simulink model "TorqueVect"  (R2022a)
settings: Solver=VariableStepAuto  StartTime=0.0  StopTime=32  RelTol=1e-3
PreLoadFcn:
  | run('Parameters\FSE_Parameters.m')
undefined symbols (not defined in the file): BRegenEnabledButton, canChannel, CyalphaLookUp, efficiency, Fz_curve, Fz_scaling_long, gearR, izz, jw, Kd, kd, Ki, ki, Kp, kp, l_f, l_r, lambda, m, Mz_max, N, N_lat, N_long, P_max, pid_kd_lat, pid_kd_long, pid_ki_lat, pid_ki_long, pid_kp_lat, pid_kp_long, R_max, rw, steerR, T_i_max, TC_Decr_Gas, TC_Derivative, TC_Incr_Gas, TC_On, TC_Relay_Off, TC_Relay_On, tireCornerStiffness, Ts, TV_On, TV_Override, velocity_lookup, velocity_lookup_lat, y_ref, yrr_scaling
libraries: simulink x218, slpidlib x135, CarMaker4SL x101, TractionControlLibrary x13, canmsglib x9, canlib x8, TorqueVectoringLibrary x6, simulink_extras x4, PedalConversionLibrary x3, PowerControlLibrary x1
(part 3 of 26)

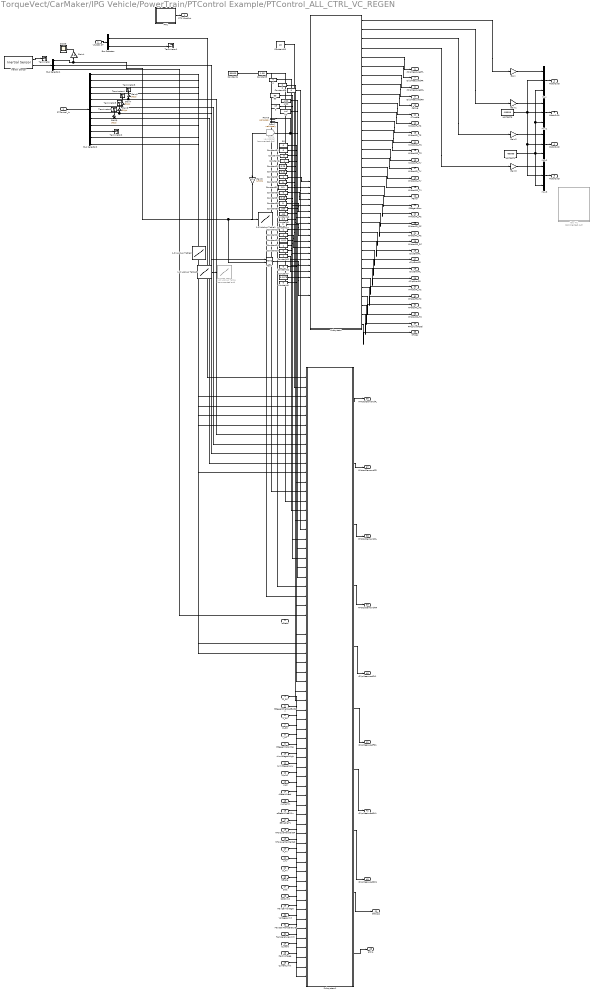
== system TorqueVect/CarMaker/IPG Vehicle/PowerTrain/PTControl Example/PTControl_ALL_CTRL_VC_REGEN ==
  VhclCtrl.PT : Inport
  PTControl_In : Inport  Port=2
  aSteer : Inport  Port=3
  FF_RC : Inport  Port=4
  BRegenEnabledButton : Inport  Port=5
  P_RC : Inport  Port=6
  D_RC : Inport  Port=7
  I_RC : Inport  Port=8
  MRegenMotorMax : Inport  Port=9
  rLimitRegenHigh : Inport  Port=10
  rLimitRegenLow : Inport  Port=11
  rSplitF : Inport  Port=12
  vLat : Inport  Port=13
  rSteerWheel : Inport  Port=14
  vLongMin : Inport  Port=15
  aSteerWheelMin : Inport  Port=16
  BEnableTV : Inport  Port=17
  NTorqueMaxDeltaF : Inport  Port=18
  NTorqueMaxDeltaR : Inport  Port=19
  P_TV : Inport  Port=20
  I_TV : Inport  Port=21
  D_TV : Inport  Port=22
  NBrake : Inport  Port=23
  Current : Inport  Port=24
  PackVoltage : Inport  Port=25
  CurrentLimit : Inport  Port=26
  SOC : Inport  Port=27
  SOClimit : Inport  Port=28
  MaxCellVoltage : Inport  Port=29
  VoltageLimit : Inport  Port=30
  MaxCellTemperature : Inport  Port=31
  TemperatureLimit : Inport  Port=32
  -20 : Constant  Value=-inf
  -200 : Constant  Value=-200
  1-D Lookup Table : Lookup_n-D  Commented=on  NumberOfTableDimensions=1  BreakpointsForDimension1=[0 5 10 15 20]  Table=[0.3 0.3 0.3 0.3 0.3]  ExtrapMethod=Clip  InternalRulePriority=Speed  RndMeth=Simplest
  1-D Lookup Table1 : Lookup_n-D  NumberOfTableDimensions=1  BreakpointsForDimension1=[-1 -0.75 -0.5 -0.25 0 0.25 0.5 0.75 1]  Table=[0.75 0.65 0.58 0.525 0.5 0.475 0.42 0.3 0.2]  ExtrapMethod=Clip  InternalRulePriority=Speed  RndMeth=Simplest
  1-D Lookup Table2 : Lookup_n-D  NumberOfTableDimensions=1  BreakpointsForDimension1=[0 5 10]  Table=[0.1 0.4 0.4]  ExtrapMethod=Clip  InternalRulePriority=Speed  RndMeth=Simplest
  1-D Lookup Table3 : Lookup_n-D  NumberOfTableDimensions=1  BreakpointsForDimension1=[0 5 10 15 20]  Table=[0.1 0.3 0.42 0.475 0.5]  ExtrapMethod=Clip  InternalRulePriority=Speed  RndMeth=Simplest
  2 : Constant  Value=2
  3 : Constant  Value=inf
  30 : Constant  Value=0
  4 : Constant  Value=4
  80 : Constant  Value=80
  Atan2 : Trigonometry  Operator=atan2
  Bus Selector : BusSelector  OutputSignals=VhclCtrl Gas,VhclCtrl Brake
  Bus Selector1 : BusSelector  OutputSignals=Vel_B x,Vel_B y,Omega_B z
  Bus Selector2 : BusSelector  OutputSignals=PT:Motor.PT:Motor:Trq,PT:Motor.PT:Motor1:Trq,PT:Motor.PT:Motor2:Trq,PT:Motor.PT:Motor3:Trq,PT:Motor.PT:Motor:rotv,PT:Motor.PT:Motor1:rotv,PT:Motor.PT:Motor2:rotv,PT:Motor.PT:Motor3:rotv,PT:PwrSupply:HV1:Pwr,Steer.Driver:Steer:Ang,Steer.Car:SteerAngle:FL,Steer.Car:SteerAngle:FR
  Constant10 : Constant  Value=18
  Constant{6,11,24,27} (4 alike) : Constant
  Constant{3,12,18,26,30..31,34,36} (8 alike) : Constant  Value=0
  Constant14 : Constant  Value=2
  Constant15 : Constant  Value=2
  Constant21 : Constant  Value=4
  Constant22 : Constant  Value=0.25
  Constant23 : Constant  Value=0.01
  Constant33 : Constant  Value=0.25
  Constant35 : Constant  Value=0.1
  Constant37 : Constant  Value=0.15
  Constant38 : Constant  Value=5
  Constant39 : Constant  Value=200
  Constant4 : Constant  Value=80000
  Constant40 : Constant  Value=-60
  Constant5 : Constant  Value=1.05
  Constant7 : Constant  Value=0.1975
  Constant9 : Constant  Value=0.5
  From4 : From  Commented=on  GotoTag=yawVelCar  TagVisibility=global
  Gain{,1..3} (4 alike) : Gain  Gain=1/21
  Gain4 : Gain  Gain=3.6
  Gain5 : Gain  Gain=1/9.81
  Gain{6..9} (4 alike) : Gain  Gain=30/pi
  Inertial Sensor : CarMaker4SL/Sensors/Inertial Sensor  xname=Param_B00  xstime=Continuous
      settings: SourceProductName=CarMaker4SL
  Mux{,1..3} (4 alike) : Mux  Inputs=3
  NOTSET1 : Constant  Value=-99999
  NOTSET3 : Constant  Value=-99999
  New TC : Subsystem  Commented=on
  PTC : Subsystem
  Scope : Scope
  Subsystem : Subsystem
  Subsystem1 : Subsystem
  Terminator{,1..6} (7 alike) : Terminator
  PTC MiscOut : Outport  VectorParamsAs1DForOutWhenUnconnected=off
  MotorOut0 : Outport  Port=2  VectorParamsAs1DForOutWhenUnconnected=off
  MotorOut1 : Outport  Port=3  VectorParamsAs1DForOutWhenUnconnected=off
  MotorOut2 : Outport  Port=4  VectorParamsAs1DForOutWhenUnconnected=off
  MotorOut3 : Outport  Port=5  VectorParamsAs1DForOutWhenUnconnected=off
  rSlipMeasuredFL : Outport  Port=6
  rSlipMeasuredFR : Outport  Port=7
  rSlipMeasuredRL : Outport  Port=8
  rSlipMeasuredRR : Outport  Port=9
  debug : Outport  Port=10
  rThrottle : Outport  Port=11
  MMotorFL_TS : Outport  Port=12
  MMotorFR_TS : Outport  Port=13
  MMotorRL_TS : Outport  Port=14
  MMotorRR_TS : Outport  Port=15
  MMotorFL_TV : Outport  Port=16
  MMotorFR_TV : Outport  Port=17
  MMotorRL_TV : Outport  Port=18
  MMotorRR_TV : Outport  Port=19
  PError : Outport  Port=20
  PRegenError : Outport  Port=21
  MMotorFL_PC : Outport  Port=22
  MMotorFR_PC : Outport  Port=23
  MMotorRL_PC : Outport  Port=24
  MMotorRR_PC : Outport  Port=25
  rSlipErrorFL : Outport  Port=26
  rSlipErrorFR : Outport  Port=27
  rSlipErrorRL : Outport  Port=28
  rSlipErrorRR : Outport  Port=29
  MMotorFL_TC : Outport  Port=30
  MMotorFR_TC : Outport  Port=31
  MMotorRL_TC : Outport  Port=32
  MMotorRR_TC : Outport  Port=33
  PPositiveTotal : Outport  Port=34
  PTotal : Outport  Port=35
  MMotorDemandFL : Outport  Port=36
  MMotorDemandFR : Outport  Port=37
  MMotorDemandRL : Outport  Port=38
  MMotorDemandRR : Outport  Port=39
  rSlipMeasuredFL1 : Outport  Port=40
  rSlipMeasuredFR1 : Outport  Port=41
  rSlipMeasuredRL1 : Outport  Port=42
  rSlipMeasuredRR1 : Outport  Port=43
  debug1 : Outport  Port=44
  aSlip : Outport  Port=45
  wires:
  VhclCtrl.PT/1 -> Bus Selector/1
  PTC/1(PTC MiscOut) -> PTC MiscOut/1
  Inertial Sensor/2 -> Bus Selector1/1
  Bus Selector1/1 -> Subsystem1/24(vLong), Atan2/2, Gain4/1  "<Vel_B x>"
  Inertial Sensor/1 -> Terminator/1
  Mux/1 -> MotorOut0/1
  Mux3/1 -> MotorOut3/1
  Mux2/1 -> MotorOut2/1
  Mux1/1 -> MotorOut1/1
  NOTSET3/1 -> Mux/2, Mux3/2, Mux2/2, Mux1/2
  NOTSET1/1 -> Mux/3, Mux1/3, Mux3/3, Mux2/3  "rotv_trg"
  Gain/1 -> Mux/1
  Gain1/1 -> Mux1/1
  Gain2/1 -> Mux2/1
  Gain3/1 -> Mux3/1
  Gain4/1 -> Scope/1
  3/1 -> Subsystem1/20(rLimitThrottleHigh)
  Constant6/1 -> Subsystem1/33(FF_TC)
  PTControl_In/1 -> Bus Selector2/1
  Subsystem/1(MMotorDemandFL) -> Gain/1
  Subsystem/2(MMotorDemandFR) -> Gain1/1
  Subsystem/3(MMotorDemandRL) -> Gain2/1
  Subsystem/4(MMotorDemandRR) -> Gain3/1
  Bus Selector2/1 -> Subsystem1/4(MMotorFR)  "<PT:Motor:Trq>"
  Bus Selector2/2 -> Subsystem1/3(MMotorFL)  "<PT:Motor1:Trq>"
  Bus Selector2/3 -> Subsystem1/5(MMotorRL)  "<PT:Motor2:Trq>"
  Bus Selector2/4 -> Subsystem1/6(MMotorRR)  "<PT:Motor3:Trq>"
  Bus Selector2/9 -> Subsystem1/11(PMeasured)  "<PT:PwrSupply:HV1:Pwr>"
  Constant11/1 -> Subsystem/43(BTVEnable)
  Constant12/1 -> Subsystem1/25(BEnableTC)
  Bus Selector2/5 -> Subsystem1/7(nMotorFL), Gain6/1  "<PT:Motor:rotv>"
  Bus Selector2/6 -> Subsystem1/8(nMotorFR), Gain7/1  "<PT:Motor1:rotv>"
  Bus Selector2/7 -> Subsystem1/9(nMotorRL), Gain8/1  "<PT:Motor2:rotv>"
  Bus Selector2/8 -> Subsystem1/10(nMotorRR), Gain9/1  "<PT:Motor3:rotv>"
  Constant14/1 -> Subsystem/37(NTorqueMaxDeltaF)
  Constant15/1 -> Subsystem/38(NTorqueMaxDeltaR)
  Bus Selector2/10 -> Terminator2/1  "<Driver:Steer:Ang>"
  Constant18/1 -> Subsystem/42(BRegenEnable)
  Constant23/1 -> Subsystem/40(I_TV)
  Constant24/1 -> Subsystem/41(D_TV)
  Constant21/1 -> Subsystem/39(P_TV)
  Bus Selector/2 -> Terminator1/1  "<VhclCtrl Brake>"
  Bus Selector1/2 -> Atan2/1  "<Vel_B y>"
  Bus Selector/1 -> Subsystem1/1(rThrottlePedal)  "<VhclCtrl Gas>"
  Bus Selector1/3 -> Subsystem1/26(nYaw)  "<Omega_B z>"
  Bus Selector2/11 -> Subsystem1/30(aSteerFL)  "<Car:SteerAngle:FL>"
  Bus Selector2/12 -> Subsystem1/29(aSteerFR)  "<Car:SteerAngle:FR>"
  Subsystem/6(rSlipMeasuredFR) -> rSlipMeasuredFR/1
  Subsystem/25(rSlipErrorFL) -> rSlipErrorFL/1
  Subsystem/30(MMotorFR_TC) -> MMotorFR_TC/1
  Atan2/1 -> Subsystem/44(aSlip)
  Subsystem/14(MMotorRR_TS) -> MMotorRR_TS/1
  Subsystem/28(rSlipErrorRR) -> rSlipErrorRR/1
  Subsystem/31(MMotorRL_TC) -> MMotorRL_TC/1
  Subsystem/26(rSlipErrorFR) -> rSlipErrorFR/1
  Subsystem/19(PError) -> PError/1
  Subsystem/23(MMotorRL_PC) -> MMotorRL_PC/1
  Subsystem/16(MMotorFR_TV) -> MMotorFR_TV/1
  Subsystem/24(MMotorRR_PC) -> MMotorRR_PC/1
  Subsystem/29(MMotorFL_TC) -> MMotorFL_TC/1
  Subsystem/32(MMotorRR_TC) -> MMotorRR_TC/1
  Subsystem/8(rSlipMeasuredRR) -> rSlipMeasuredRR/1
  Subsystem/12(MMotorFR_TS) -> MMotorFR_TS/1
  Subsystem/34(PTotal) -> PTotal/1
  Subsystem/10(rThrottle) -> rThrottle/1
  Subsystem/21(MMotorFL_PC) -> MMotorFL_PC/1
  Subsystem/15(MMotorFL_TV) -> MMotorFL_TV/1
  Constant4/1 -> Subsystem1/13(PLimit)
  Subsystem/7(rSlipMeasuredRL) -> rSlipMeasuredRL/1
  Subsystem/20(PRegenError) -> PRegenError/1
  Subsystem/22(MMotorFR_PC) -> MMotorFR_PC/1
  Subsystem/9(debug) -> debug/1
  Subsystem/5(rSlipMeasuredFL) -> rSlipMeasuredFL/1
  Subsystem/18(MMotorRR_TV) -> MMotorRR_TV/1
  Constant5/1 -> Subsystem1/14(FF_PC)
  Constant10/1 -> Subsystem1/2(MMotorMax)
  Subsystem/13(MMotorRL_TS) -> MMotorRL_TS/1
  Subsystem/11(MMotorFL_TS) -> MMotorFL_TS/1
  Subsystem/27(rSlipErrorRL) -> rSlipErrorRL/1
  Subsystem/17(MMotorRL_TV) -> MMotorRL_TV/1
  4/1 -> Subsystem1/15(P_PC)
  Subsystem/33(PPositiveTotal) -> PPositiveTotal/1
  2/1 -> Subsystem1/16(D_PC)
  Constant26/1 -> Subsystem1/17(I_PC)
  80/1 -> Subsystem1/18(rLimitHigh)
  -200/1 -> Subsystem1/19(rLimitLow)
  30/1 -> Subsystem1/28(P_TC)
  Constant31/1 -> Subsystem1/31(D_TC)
  Constant30/1 -> Subsystem1/32(I_TC)
  Constant22/1 -> Subsystem1/34(rSlipTargetF)
  Constant33/1 -> Subsystem1/35(rSlipTargetR)
  Constant27/1 -> Subsystem/28(FF_RC)
  Constant34/1 -> Subsystem/29(PRegenLimit)
  Constant35/1 -> Subsystem/30(P_RC)
  Constant36/1 -> Subsystem/31(D_RC)
  Constant37/1 -> Subsystem/32(I_RC)
  Constant38/1 -> Subsystem/33(MRegenMotorMax)
  Constant39/1 -> Subsystem/34(rLimitRegenHigh)
  Constant40/1 -> Subsystem/35(rLimitRegenLow)
  [vehAccelx] -> Subsystem1/22(aLong), Gain5/1
  Constant3/1 -> Subsystem1/12(BMeasuredEnable)
  -20/1 -> Subsystem1/21(rLimitThrottleLow)
  1-D Lookup Table3/1 -> 1-D Lookup Table/1
  Gain5/1 -> 1-D Lookup Table1/1
  Constant7/1 -> Subsystem/47(rWheel)
  Constant9/1 -> Subsystem/36(rSplitF)
  Gain6/1 -> Terminator3/1  "FL RPM"
  Gain8/1 -> Terminator5/1  "RL RPM"
  Gain7/1 -> Terminator4/1  "FR RPM"
  Gain9/1 -> Terminator6/1  "RR RPM"
  [vehAccely] -> Subsystem1/23(aLat)
  MaxCellVoltage/1 -> Subsystem1/58(MaxCellVoltage)
  vLongMin/1 -> Subsystem1/47(vLongMin)
  CurrentLimit/1 -> Subsystem1/64(CurrentLimit)
  NBrake/1 -> Subsystem1/55(NBrake)
  I_RC/1 -> Subsystem1/40(I_RC)
  rSteerWheel/1 -> Subsystem1/46(rSteerWheel)
  Subsystem1/4(MMotorDemandRR) -> MMotorDemandRR/1
  Subsystem1/5(rSlipMeasuredFL) -> rSlipMeasuredFL1/1
  P_RC/1 -> Subsystem1/38(P_RC)
  Current/1 -> Subsystem1/62(Current)
  BRegenEnabledButton/1 -> Subsystem1/37(BRegenEnabledButton)
  Subsystem1/3(MMotorDemandRL) -> MMotorDemandRL/1
  Subsystem1/1(MMotorDemandFL) -> MMotorDemandFL/1
  Subsystem1/7(rSlipMeasuredRL) -> rSlipMeasuredRL1/1
  Subsystem1/2(MMotorDemandFR) -> MMotorDemandFR/1
  rLimitRegenHigh/1 -> Subsystem1/42(rLimitRegenHigh)
  SOC/1 -> Subsystem1/56(SOC)
  VoltageLimit/1 -> Subsystem1/59(VoltageLimit)
  SOClimit/1 -> Subsystem1/57(SOClimit)
  MRegenMotorMax/1 -> Subsystem1/41(MRegenMotorMax)
  rLimitRegenLow/1 -> Subsystem1/43(rLimitRegenLow)
  Subsystem1/8(rSlipMeasuredRR) -> rSlipMeasuredRR1/1
  TemperatureLimit/1 -> Subsystem1/61(TemperatureLimit)
  FF_RC/1 -> Subsystem1/36(FF_RC)
  rSplitF/1 -> Subsystem1/44(rSplitF)
  aSteerWheelMin/1 -> Subsystem1/48(aSteerWheelMin)
  I_TV/1 -> Subsystem1/53(I_TV)
  NTorqueMaxDeltaF/1 -> Subsystem1/50(NTorqueMaxDeltaF)
  Subsystem1/9(debug) -> debug1/1
  Subsystem1/6(rSlipMeasuredFR) -> rSlipMeasuredFR1/1
  NTorqueMaxDeltaR/1 -> Subsystem1/51(NTorqueMaxDeltaR)
  MaxCellTemperature/1 -> Subsystem1/60(MaxCellTemperature)
  D_RC/1 -> Subsystem1/39(D_RC)
  D_TV/1 -> Subsystem1/54(D_TV)
  Subsystem1/10(aSlip) -> aSlip/1
  BEnableTV/1 -> Subsystem1/49(BTorqueVectoringEnable)
  PackVoltage/1 -> Subsystem1/63(PackVoltage)
  vLat/1 -> Subsystem1/45(vLat)
  P_TV/1 -> Subsystem1/52(P_TV)

== system TorqueVect/CarMaker/IPG Vehicle/PowerTrain/PTControl Example/PTControl_ALL_Speedgoat ==
  VhclCtrl.PT : Inport
  PTControl_In : Inport  Port=2
  Gain{,1..3} (4 alike) : Gain  Gain=1/21
  Mux{,1..3} (4 alike) : Mux  Inputs=3
  NOTSET1 : Constant  Value=-99999
  NOTSET3 : Constant  Value=-99999
  New TC : Subsystem  Commented=on
  PTC : Subsystem
  Subsystem : Subsystem
  PTC MiscOut : Outport  VectorParamsAs1DForOutWhenUnconnected=off
  MotorOut0 : Outport  Port=2  VectorParamsAs1DForOutWhenUnconnected=off
  MotorOut1 : Outport  Port=3  VectorParamsAs1DForOutWhenUnconnected=off
  MotorOut2 : Outport  Port=4  VectorParamsAs1DForOutWhenUnconnected=off
  MotorOut3 : Outport  Port=5  VectorParamsAs1DForOutWhenUnconnected=off
  wires:
  PTC/1(PTC MiscOut) -> PTC MiscOut/1
  Mux/1 -> MotorOut0/1
  Mux3/1 -> MotorOut3/1
  Mux2/1 -> MotorOut2/1
  Mux1/1 -> MotorOut1/1
  NOTSET3/1 -> Mux3/2, Mux2/2, Mux1/2, Mux/2
  NOTSET1/1 -> Mux3/3, Mux2/3, Mux/3, Mux1/3  "rotv_trg"
  Gain/1 -> Mux/1
  Gain1/1 -> Mux1/1
  Gain2/1 -> Mux2/1
  Gain3/1 -> Mux3/1
  VhclCtrl.PT/1 -> Subsystem/1(VhclCtrl.PT)
  PTControl_In/1 -> Subsystem/2(PTControl_In)
  Subsystem/1(<PT:Motor:Trq>) -> Gain/1
  Subsystem/2(<PT:Motor1:Trq>) -> Gain1/1
  Subsystem/3(<PT:Motor2:Trq>) -> Gain2/1
  Subsystem/4(<PT:Motor3:Trq>) -> Gain3/1

== system TorqueVect/CarMaker/IPG Vehicle/PowerTrain/PTControl Example/PTControl_In ==
  note: [1:43 PM] Ali (Guest)rTireSlipCombinedXX = sqrt(rTireSlipXX^2 + aTireSlipXX^2)
  Sync_In : Inport
  Add{,1..3} (4 alike) : Sum
  Bus Creator : BusCreator  Inputs=8
  Bus Creator1 : BusCreator  Inputs=4
  Bus Creator2 : BusCreator  Inputs=4
  Bus Creator3 : BusCreator  Inputs=3
  CreateBus PTControl_In : BusCreator  Inputs=4
  Read CM Dict : CarMaker4SL/Read CM Dict  xname=PT.Motor.Trq  xsync=on  xstime=Continuous
  Read CM Dict1 : CarMaker4SL/Read CM Dict  xname=PT.Motor1.Trq  xsync=on  xstime=Continuous
  Read CM Dict10 : CarMaker4SL/Read CM Dict  xname=Vhcl.FR.LongSlip  xsync=on  xstime=Continuous
  Read CM Dict11 : CarMaker4SL/Read CM Dict  xname=Vhcl.RL.LongSlip  xsync=on  xstime=Continuous
  Read CM Dict12 : CarMaker4SL/Read CM Dict  xname=Vhcl.RR.LongSlip  xsync=on  xstime=Continuous
  Read CM Dict13 : CarMaker4SL/Read CM Dict  xname=Driver.Steer.Ang  xsync=on  xstime=Continuous
  Read CM Dict14 : CarMaker4SL/Read CM Dict  xname=Vhcl.FR.LongSlip  xsync=on  xstime=Continuous
  Read CM Dict15 : CarMaker4SL/Read CM Dict  xname=Vhcl.RL.LongSlip  xsync=on  xstime=Continuous
  Read CM Dict16 : CarMaker4SL/Read CM Dict  xname=Vhcl.RR.LongSlip  xsync=on  xstime=Continuous
  Read CM Dict17 : CarMaker4SL/Read CM Dict  xname=Vhcl.FL.LongSlip  xsync=on  xstime=Continuous
  Read CM Dict18 : CarMaker4SL/Read CM Dict  xname=Vhcl.FR.SideSlip  xsync=on  xstime=Continuous
  Read CM Dict19 : CarMaker4SL/Read CM Dict  xname=Vhcl.RL.SideSlip  xsync=on  xstime=Continuous
  Read CM Dict2 : CarMaker4SL/Read CM Dict  xname=PT.Motor2.Trq  xsync=on  xstime=Continuous
  Read CM Dict20 : CarMaker4SL/Read CM Dict  xname=Vhcl.RR.SideSlip  xsync=on  xstime=Continuous
  Read CM Dict21 : CarMaker4SL/Read CM Dict  xname=Vhcl.FL.SideSlip  xsync=on  xstime=Continuous
  Read CM Dict22 : CarMaker4SL/Read CM Dict  xname=Car.SteerAngleFL  xsync=on  xstime=Continuous
  Read CM Dict23 : CarMaker4SL/Read CM Dict  xname=Car.SteerAngleFR  xsync=on  xstime=Continuous
  Read CM Dict24 : CarMaker4SL/Read CM Dict  xname=Car.WFL.Radius  xsync=on  xstime=Continuous
  Read CM Dict3 : CarMaker4SL/Read CM Dict  xname=PT.Motor3.Trq  xsync=on  xstime=Continuous
  Read CM Dict4 : CarMaker4SL/Read CM Dict  xname=PT.Motor.rotv  xsync=on  xstime=Continuous
  Read CM Dict5 : CarMaker4SL/Read CM Dict  xname=PT.Motor1.rotv  xsync=on  xstime=Continuous
  Read CM Dict6 : CarMaker4SL/Read CM Dict  xname=PT.Motor2.rotv  xsync=on  xstime=Continuous
  Read CM Dict7 : CarMaker4SL/Read CM Dict  xname=PT.Motor3.rotv  xsync=on  xstime=Continuous
  Read CM Dict8 : CarMaker4SL/Read CM Dict  xname=PT.PwrSupply.HV1.Pwr  xsync=on  xstime=Continuous
  Read CM Dict9 : CarMaker4SL/Read CM Dict  xname=Vhcl.FL.LongSlip  xsync=on  xstime=Continuous
  Sqrt{,1..3} (4 alike) : Sqrt
  Square{,1..7} (8 alike) : Math  Operator=square
  Terminator : Terminator
  Terminator1 : Terminator
  PTControl_In : Outport  VectorParamsAs1DForOutWhenUnconnected=off
  wires:
  Sync_In/1 -> Read CM Dict2/1, Read CM Dict/1, Read CM Dict1/1, Read CM Dict22/1, Read CM Dict23/1, Read CM Dict21/1, Read CM Dict14/1, Read CM Dict24/1, Read CM Dict20/1, Read CM Dict16/1, Read CM Dict19/1, Read CM Dict15/1, Read CM Dict18/1, Read CM Dict17/1, Read CM Dict13/1, Read CM Dict12/1, Read CM Dict11/1, Read CM Dict10/1, Read CM Dict9/1, Read CM Dict8/1, Read CM Dict7/1, Read CM Dict6/1, Read CM Dict5/1, Read CM Dict4/1, Read CM Dict3/1
  CreateBus PTControl_In/1 -> PTControl_In/1
  Read CM Dict/1 -> Bus Creator/1  "PT.Motor.Trq"
  Read CM Dict1/1 -> Bus Creator/2  "PT.Motor1.Trq"
  Read CM Dict2/1 -> Bus Creator/3  "PT.Motor2.Trq"
  Read CM Dict3/1 -> Bus Creator/4  "PT.Motor3.Trq"
  Read CM Dict4/1 -> Bus Creator/5  "PT.Motor.rotv"
  Read CM Dict5/1 -> Bus Creator/6  "PT.Motor1.rotv"
  Read CM Dict6/1 -> Bus Creator/7  "PT.Motor2.rotv"
  Read CM Dict7/1 -> Bus Creator/8  "PT.Motor3.rotv"
  Bus Creator/1 -> CreateBus PTControl_In/1  "PT.Motor"
  Read CM Dict8/1 -> CreateBus PTControl_In/2  "PT.PwrSupply.HV1.Pwr"
  Read CM Dict12/1 -> Bus Creator1/4  "Vhcl.RR.LongSlip"
  Read CM Dict11/1 -> Bus Creator1/3  "Vhcl.RL.LongSlip"
  Read CM Dict10/1 -> Bus Creator1/2  "Vhcl.FR.LongSlip"
  Read CM Dict9/1 -> Bus Creator1/1  "Vhcl.FL.LongSlip"
  Bus Creator1/1 -> CreateBus PTControl_In/3  "VhclTyres"
  Read CM Dict17/1 -> Square/1  "Vhcl.FL.LongSlip"
  Read CM Dict21/1 -> Square1/1  "Vhcl.FL.LongSlip"
  Read CM Dict14/1 -> Square2/1  "Vhcl.FR.LongSlip"
  Read CM Dict18/1 -> Square3/1  "Vhcl.FR.LongSlip"
  Read CM Dict15/1 -> Square4/1  "Vhcl.RL.LongSlip"
  Read CM Dict19/1 -> Square5/1  "Vhcl.RL.LongSlip"
  Read CM Dict16/1 -> Square6/1  "Vhcl.RR.LongSlip"
  Read CM Dict20/1 -> Square7/1  "Vhcl.RR.LongSlip"
  Square/1 -> Add/1
  Square1/1 -> Add/2
  Square2/1 -> Add1/1
  Square3/1 -> Add1/2
  Square5/1 -> Add2/2
  Square4/1 -> Add2/1
  Square6/1 -> Add3/1
  Square7/1 -> Add3/2
  Add/1 -> Sqrt/1
  Add1/1 -> Sqrt1/1
  Add2/1 -> Sqrt2/1
  Add3/1 -> Sqrt3/1
  Sqrt/1 -> Bus Creator2/1  "FL"
  Sqrt1/1 -> Bus Creator2/2  "FR"
  Sqrt2/1 -> Bus Creator2/3  "RL"
  Sqrt3/1 -> Bus Creator2/4  "RR"
  Bus Creator2/1 -> Terminator/1  "combined"
  Bus Creator3/1 -> CreateBus PTControl_In/4  "Steer"
  Read CM Dict13/1 -> Bus Creator3/1  "Driver.Steer.Ang"
  Read CM Dict22/1 -> Bus Creator3/2  "Car.SteerAngle.FL"
  Read CM Dict23/1 -> Bus Creator3/3  "Car.SteerAngle.FR"
  Read CM Dict24/1 -> Terminator1/1  "FL_radius"

== system TorqueVect/CarMaker/IPG Vehicle/PowerTrain/PTControl Example/PTControl_In1 ==
  Sync_In : Inport
  CreateBus PTC Battery : Subsystem
  CreateBus PTC ClutchIn : Subsystem
  CreateBus PTC Control Units : Subsystem
  CreateBus PTC DriveSrcIn : Subsystem
  CreateBus PTC EngineIn : Subsystem
  CreateBus PTC GearBoxIn : Subsystem
  CreateBus PTC GearBoxM_In0 : Subsystem
  CreateBus PTC GearBoxM_In1 : Subsystem
  CreateBus PTC GearBoxM_In2 : Subsystem
  CreateBus PTC GearBoxM_In3 : Subsystem
  CreateBus PTC ISGIn : Subsystem
  CreateBus PTC MotorIn0 : Subsystem
  CreateBus PTC MotorIn1 : Subsystem
  CreateBus PTC MotorIn2 : Subsystem
  CreateBus PTC MotorIn3 : Subsystem
  CreateBus PTC PwrSupplyIn : Subsystem
  CreateBus PTC Vehicle Ctrl : Subsystem
  CreateBus PTC WheelIn : Subsystem
  CreateBus PTC_Cfg Battery : Subsystem
  CreateBus PTC_Cfg Engine : Subsystem
  CreateBus PTC_Cfg GearBox : Subsystem
  CreateBus PTC_Cfg GearBoxM0 : Subsystem
  CreateBus PTC_Cfg GearBoxM1 : Subsystem
  CreateBus PTC_Cfg GearBoxM2 : Subsystem
  CreateBus PTC_Cfg GearBoxM3 : Subsystem
  CreateBus PTC_Cfg ISG : Subsystem
  CreateBus PTC_Cfg Misc : Subsystem
  CreateBus PTC_Cfg Motor : Subsystem
  CreateBus PTC_Cfg PlanetGear : Subsystem
  CreateBus PTControl_In : BusCreator  Inputs=29
  S-Function : S-Function  FunctionName=cm_ptcontrol_in  SFunctionDeploymentMode=off  EnableBusSupport=off
  PTControl_In : Outport  VectorParamsAs1DForOutWhenUnconnected=off
  wires:
  Sync_In/1 -> S-Function/1
  CreateBus PTControl_In/1 -> PTControl_In/1
  S-Function/1 -> CreateBus PTC_Cfg Misc/1(In)
  CreateBus PTC_Cfg Misc/1(Out) -> CreateBus PTControl_In/1  "PTC_Cfg Misc"
  S-Function/2 -> CreateBus PTC_Cfg Battery/1(In)
  CreateBus PTC_Cfg Battery/1(Out) -> CreateBus PTControl_In/2  "PTC_Cfg Battery"
  S-Function/3 -> CreateBus PTC_Cfg Engine/1(In)
  CreateBus PTC_Cfg Engine/1(Out) -> CreateBus PTControl_In/3  "PTC_Cfg Engine"
  S-Function/4 -> CreateBus PTC_Cfg ISG/1(In)
  CreateBus PTC_Cfg ISG/1(Out) -> CreateBus PTControl_In/4  "PTC_Cfg ISG"
  S-Function/5 -> CreateBus PTC_Cfg Motor/1(In)
  CreateBus PTC_Cfg Motor/1(Out) -> CreateBus PTControl_In/5  "PTC_Cfg Motor"
  S-Function/6 -> CreateBus PTC_Cfg GearBox/1(In)
  CreateBus PTC_Cfg GearBox/1(Out) -> CreateBus PTControl_In/6  "PTC_Cfg GearBox"
  S-Function/7 -> CreateBus PTC_Cfg GearBoxM0/1(In)
  CreateBus PTC_Cfg GearBoxM0/1(Out) -> CreateBus PTControl_In/7  "PTC_Cfg GearBoxM0"
  S-Function/8 -> CreateBus PTC_Cfg GearBoxM1/1(In)
  CreateBus PTC_Cfg GearBoxM1/1(Out) -> CreateBus PTControl_In/8  "PTC_Cfg GearBoxM1"
  S-Function/9 -> CreateBus PTC_Cfg GearBoxM2/1(In)
  CreateBus PTC_Cfg GearBoxM2/1(Out) -> CreateBus PTControl_In/9  "PTC_Cfg GearBoxM2"
  S-Function/10 -> CreateBus PTC_Cfg GearBoxM3/1(In)
  CreateBus PTC_Cfg GearBoxM3/1(Out) -> CreateBus PTControl_In/10  "PTC_Cfg GearBoxM3"
  S-Function/11 -> CreateBus PTC_Cfg PlanetGear/1(In)
  CreateBus PTC_Cfg PlanetGear/1(Out) -> CreateBus PTControl_In/11  "PTC_Cfg PlanetGear"
  S-Function/12 -> CreateBus PTC Vehicle Ctrl/1(In)
  CreateBus PTC Vehicle Ctrl/1(Out) -> CreateBus PTControl_In/12  "PTC Vehicle Ctrl"
  S-Function/13 -> CreateBus PTC Control Units/1(In)
  CreateBus PTC Control Units/1(Out) -> CreateBus PTControl_In/13  "PTC Control Units"
  S-Function/14 -> CreateBus PTC EngineIn/1(In)
  CreateBus PTC EngineIn/1(Out) -> CreateBus PTControl_In/14  "PTC EngineIn"
  S-Function/15 -> CreateBus PTC ISGIn/1(In)
  CreateBus PTC ISGIn/1(Out) -> CreateBus PTControl_In/15  "PTC ISGIn"
  S-Function/16 -> CreateBus PTC MotorIn0/1(In)
  CreateBus PTC MotorIn0/1(Out) -> CreateBus PTControl_In/16  "PTC MotorIn0"
  S-Function/17 -> CreateBus PTC MotorIn1/1(In)
  CreateBus PTC MotorIn1/1(Out) -> CreateBus PTControl_In/17  "PTC MotorIn1"
  S-Function/18 -> CreateBus PTC MotorIn2/1(In)
  CreateBus PTC MotorIn2/1(Out) -> CreateBus PTControl_In/18  "PTC MotorIn2"
  S-Function/19 -> CreateBus PTC MotorIn3/1(In)
  CreateBus PTC MotorIn3/1(Out) -> CreateBus PTControl_In/19  "PTC MotorIn3"
  S-Function/20 -> CreateBus PTC ClutchIn/1(In)
  CreateBus PTC ClutchIn/1(Out) -> CreateBus PTControl_In/20  "PTC ClutchIn"
  S-Function/21 -> CreateBus PTC GearBoxIn/1(In)
  CreateBus PTC GearBoxIn/1(Out) -> CreateBus PTControl_In/21  "PTC GearBoxIn"
  S-Function/22 -> CreateBus PTC GearBoxM_In0/1(In)
  CreateBus PTC GearBoxM_In0/1(Out) -> CreateBus PTControl_In/22  "PTC GearBoxM_In0"
  S-Function/23 -> CreateBus PTC GearBoxM_In1/1(In)
  CreateBus PTC GearBoxM_In1/1(Out) -> CreateBus PTControl_In/23  "PTC GearBoxM_In1"
  S-Function/24 -> CreateBus PTC GearBoxM_In2/1(In)
  CreateBus PTC GearBoxM_In2/1(Out) -> CreateBus PTControl_In/24  "PTC GearBoxM_In2"
  S-Function/25 -> CreateBus PTC GearBoxM_In3/1(In)
  CreateBus PTC GearBoxM_In3/1(Out) -> CreateBus PTControl_In/25  "PTC GearBoxM_In3"
  S-Function/26 -> CreateBus PTC Battery/1(In)
  CreateBus PTC Battery/1(Out) -> CreateBus PTControl_In/26  "PTC Battery"
  S-Function/27 -> CreateBus PTC PwrSupplyIn/1(In)
  CreateBus PTC PwrSupplyIn/1(Out) -> CreateBus PTControl_In/27  "PTC PwrSupplyIn"
  S-Function/28 -> CreateBus PTC WheelIn/1(In)
  CreateBus PTC WheelIn/1(Out) -> CreateBus PTControl_In/28  "PTC WheelIn"
  S-Function/29 -> CreateBus PTC DriveSrcIn/1(In)
  CreateBus PTC DriveSrcIn/1(Out) -> CreateBus PTControl_In/29  "PTC DriveSrcIn"

== system TorqueVect/CarMaker/IPG Vehicle/PowerTrain/PTControl Example/PTControl_Out ==
  PTC MiscOut : Inport
  PTC EngineOut : Inport  Port=2
  PTC ISGOut : Inport  Port=3
  PTC MotorOut0 : Inport  Port=4
  PTC MotorOut1 : Inport  Port=5
  PTC MotorOut2 : Inport  Port=6
  PTC MotorOut3 : Inport  Port=7
  PTC ClutchOut : Inport  Port=8
  PTC GearBoxOut : Inport  Port=9
  PTC GearBoxM_Out0 : Inport  Port=10
  PTC GearBoxM_Out1 : Inport  Port=11
  PTC GearBoxM_Out2 : Inport  Port=12
  PTC GearBoxM_Out3 : Inport  Port=13
  PTC PwrSupplyOut : Inport  Port=14
  PTC WheelOut : Inport  Port=15
  PTControl_Out : S-Function  FunctionName=cm_ptcontrol_out  SFunctionDeploymentMode=off  EnableBusSupport=off
  wires:
  PTC MiscOut/1 -> PTControl_Out/1
  PTC EngineOut/1 -> PTControl_Out/2
  PTC ISGOut/1 -> PTControl_Out/3
  PTC MotorOut0/1 -> PTControl_Out/4
  PTC MotorOut1/1 -> PTControl_Out/5
  PTC MotorOut2/1 -> PTControl_Out/6
  PTC MotorOut3/1 -> PTControl_Out/7
  PTC ClutchOut/1 -> PTControl_Out/8
  PTC GearBoxOut/1 -> PTControl_Out/9
  PTC GearBoxM_Out0/1 -> PTControl_Out/10
  PTC GearBoxM_Out1/1 -> PTControl_Out/11
  PTC GearBoxM_Out2/1 -> PTControl_Out/12
  PTC GearBoxM_Out3/1 -> PTControl_Out/13
  PTC PwrSupplyOut/1 -> PTControl_Out/14
  PTC WheelOut/1 -> PTControl_Out/15

== system TorqueVect/CarMaker/IPG Vehicle/PowerTrain/PTControl Example/PTControl_PC_MFE ==
  VhclCtrl.PT : Inport
  PTControl_In : Inport  Port=2
  Bus Selector : BusSelector  OutputSignals=VhclCtrl Gas
  Bus Selector1 : BusSelector  OutputSignals=Vel_B x
  Bus Selector2 : BusSelector  OutputSignals=PT:Motor.PT:Motor:Trq,PT:Motor.PT:Motor1:Trq,PT:Motor.PT:Motor2:Trq,PT:Motor.PT:Motor3:Trq,PT:Motor.PT:Motor:rotv,PT:Motor.PT:Motor1:rotv,PT:Motor.PT:Motor2:rotv,PT:Motor.PT:Motor3:rotv,PT:PwrSupply:HV1:Pwr
  Constant : Constant
  Constant1 : Constant  Value=0.4
  Constant10 : Constant  Value=14
  Constant2 : Constant  Value=0.6
  Constant3 : Constant  Value=10000
  Constant4 : Constant  Value=40000
  Constant5 : Constant  Value=1.05
  Constant6 : Constant  Value=1.05
  Constant7 : Constant  Value=12
  Constant8 : Constant  Value=0
  Constant9 : Constant  Value=7
  Gain{,1..3} (4 alike) : Gain  Gain=1/21
  Gain4 : Gain  Gain=3.6
  Inertial Sensor : CarMaker4SL/Sensors/Inertial Sensor  xname=Param_B00  xstime=Continuous
      settings: SourceProductName=CarMaker4SL
  Mux{,1..3} (4 alike) : Mux  Inputs=3
  NOTSET1 : Constant  Value=-99999
  NOTSET3 : Constant  Value=-99999
  New TC : Subsystem  Commented=on
  PTC : Subsystem
  Scope : Scope
  Subsystem : Subsystem
  Terminator : Terminator
  PTC MiscOut : Outport  VectorParamsAs1DForOutWhenUnconnected=off
  MotorOut0 : Outport  Port=2  VectorParamsAs1DForOutWhenUnconnected=off
  MotorOut1 : Outport  Port=3  VectorParamsAs1DForOutWhenUnconnected=off
  MotorOut2 : Outport  Port=4  VectorParamsAs1DForOutWhenUnconnected=off
  MotorOut3 : Outport  Port=5  VectorParamsAs1DForOutWhenUnconnected=off
  wires:
  VhclCtrl.PT/1 -> Bus Selector/1
  PTC/1(PTC MiscOut) -> PTC MiscOut/1
  Inertial Sensor/2 -> Bus Selector1/1
  Bus Selector1/1 -> Subsystem/2(vLong), Gain4/1  "<Vel_B x>"
  Inertial Sensor/1 -> Terminator/1
  Mux/1 -> MotorOut0/1
  Mux3/1 -> MotorOut3/1
  Mux2/1 -> MotorOut2/1
  Mux1/1 -> MotorOut1/1
  NOTSET3/1 -> Mux3/2, Mux1/2, Mux/2, Mux2/2
  NOTSET1/1 -> Mux/3, Mux1/3, Mux2/3, Mux3/3  "rotv_trg"
  Gain/1 -> Mux/1
  Gain1/1 -> Mux1/1
  Gain2/1 -> Mux2/1
  Gain3/1 -> Mux3/1
  Bus Selector/1 -> Subsystem/1(rThrottlePedal)  "<VhclCtrl Gas>"
  Gain4/1 -> Scope/1
  Subsystem/1(MMotorDemandFL) -> Gain/1
  Subsystem/2(MMotorDemandFR) -> Gain1/1
  Subsystem/3(MMotorDemandRL) -> Gain2/1
  Subsystem/4(MMotorDemandRR) -> Gain3/1
  Constant8/1 -> Subsystem/3(BRegenEnabledButton)
  Constant/1 -> Subsystem/13(BMeasuredEnable)
  Constant1/1 -> Subsystem/14(rSplitF)
  Constant2/1 -> Subsystem/15(rRegenSplitF)
  Constant3/1 -> Subsystem/16(PRegenLimit)
  Constant4/1 -> Subsystem/17(PLimit)
  Constant5/1 -> Subsystem/18(FF_PC)
  Constant6/1 -> Subsystem/19(FF_RC)
  Constant7/1 -> Subsystem/20(P_PC)
  Constant9/1 -> Subsystem/21(D_PC)
  Constant10/1 -> Subsystem/22(MMotorMax)
  Bus Selector2/1 -> Subsystem/4(MMotorFL)  "<PT:Motor:Trq>"
  Bus Selector2/2 -> Subsystem/5(MMotorFR)  "<PT:Motor1:Trq>"
  Bus Selector2/3 -> Subsystem/6(MMotorRL)  "<PT:Motor2:Trq>"
  Bus Selector2/4 -> Subsystem/7(MMotorRR)  "<PT:Motor3:Trq>"
  Bus Selector2/7 -> Subsystem/10(nMotorRL)  "<PT:Motor2:rotv>"
  Bus Selector2/8 -> Subsystem/11(nMotorRR)  "<PT:Motor3:rotv>"
  Bus Selector2/5 -> Subsystem/8(nMotorFL)  "<PT:Motor:rotv>"
  Bus Selector2/6 -> Subsystem/9(nMotorFR)  "<PT:Motor1:rotv>"
  Bus Selector2/9 -> Subsystem/12(PMeasured)  "<PT:PwrSupply:HV1:Pwr>"
  PTControl_In/1 -> Bus Selector2/1

== system TorqueVect/CarMaker/IPG Vehicle/PowerTrain/PTControl Example/PTControl_PC_TC_MFE ==
  VhclCtrl.PT : Inport
  PTControl_In : Inport  Port=2
  Bus Selector : BusSelector  OutputSignals=VhclCtrl Gas
  Bus Selector1 : BusSelector  OutputSignals=Vel_B x
  Bus Selector2 : BusSelector  OutputSignals=PT:Motor.PT:Motor:Trq,PT:Motor.PT:Motor1:Trq,PT:Motor.PT:Motor2:Trq,PT:Motor.PT:Motor3:Trq,PT:Motor.PT:Motor:rotv,PT:Motor.PT:Motor1:rotv,PT:Motor.PT:Motor2:rotv,PT:Motor.PT:Motor3:rotv,PT:PwrSupply:HV1:Pwr
  Constant{,8,11..12} (4 alike) : Constant
  Constant1 : Constant  Value=0.1
  Constant10 : Constant  Value=18
  Constant13 : Constant  Value=0.6
  Constant14 : Constant  Value=12
  Constant15 : Constant  Value=7
  Constant16 : Constant  Value=100
  Constant17 : Constant  Value=-100
  Constant2 : Constant  Value=0.4
  Constant3 : Constant  Value=10000
  Constant4 : Constant  Value=80000
  Constant5 : Constant  Value=1.05
  Constant6 : Constant  Value=1.05
  Constant7 : Constant  Value=12
  Constant9 : Constant  Value=7
  Gain{,1..3} (4 alike) : Gain  Gain=1/21
  Gain4 : Gain  Gain=3.6
  Inertial Sensor : CarMaker4SL/Sensors/Inertial Sensor  xname=Param_B00  xstime=Continuous
      settings: SourceProductName=CarMaker4SL
  Mux{,1..3} (4 alike) : Mux  Inputs=3
  NOTSET1 : Constant  Value=-99999
  NOTSET3 : Constant  Value=-99999
  New TC : Subsystem  Commented=on
  PTC : Subsystem
  Scope : Scope
  Subsystem1 : Subsystem
  Terminator : Terminator
  PTC MiscOut : Outport  VectorParamsAs1DForOutWhenUnconnected=off
  MotorOut0 : Outport  Port=2  VectorParamsAs1DForOutWhenUnconnected=off
  MotorOut1 : Outport  Port=3  VectorParamsAs1DForOutWhenUnconnected=off
  MotorOut2 : Outport  Port=4  VectorParamsAs1DForOutWhenUnconnected=off
  MotorOut3 : Outport  Port=5  VectorParamsAs1DForOutWhenUnconnected=off
  wires:
  VhclCtrl.PT/1 -> Bus Selector/1
  PTC/1(PTC MiscOut) -> PTC MiscOut/1
  Inertial Sensor/2 -> Bus Selector1/1
  Bus Selector1/1 -> Subsystem1/2(vLong), Gain4/1  "<Vel_B x>"
  Inertial Sensor/1 -> Terminator/1
  Mux/1 -> MotorOut0/1
  Mux3/1 -> MotorOut3/1
  Mux2/1 -> MotorOut2/1
  Mux1/1 -> MotorOut1/1
  NOTSET3/1 -> Mux3/2, Mux1/2, Mux/2, Mux2/2
  NOTSET1/1 -> Mux/3, Mux1/3, Mux2/3, Mux3/3  "rotv_trg"
  Gain/1 -> Mux/1
  Gain1/1 -> Mux1/1
  Gain2/1 -> Mux2/1
  Gain3/1 -> Mux3/1
  Bus Selector/1 -> Subsystem1/1(rThrottlePedal)  "<VhclCtrl Gas>"
  Gain4/1 -> Scope/1
  Constant8/1 -> Subsystem1/3(BRegenEnabledButton)
  Constant/1 -> Subsystem1/10(BEnableTC)
  Constant1/1 -> Subsystem1/9(rSlipTargetR), Subsystem1/8(rSlipTargetF)
  Constant2/1 -> Subsystem1/16(rSplitF)
  Constant3/1 -> Subsystem1/19(PRegenLimit)
  Constant4/1 -> Subsystem1/21(PLimit)
  Constant5/1 -> Subsystem1/22(FF_PC)
  Constant6/1 -> Subsystem1/23(FF_RC)
  Constant7/1 -> Subsystem1/11(P_TC)
  Constant9/1 -> Subsystem1/13(D_TC)
  Constant10/1 -> Subsystem1/26(MMotorMax)
  PTControl_In/1 -> Bus Selector2/1
  Subsystem1/1(MMotorDemandFL) -> Gain/1
  Subsystem1/2(MMotorDemandFR) -> Gain1/1
  Subsystem1/3(MMotorDemandRL) -> Gain2/1
  Subsystem1/4(MMotorDemandRR) -> Gain3/1
  Bus Selector2/1 -> Subsystem1/4(MMotorFL)  "<PT:Motor:Trq>"
  Bus Selector2/2 -> Subsystem1/5(MMotorFR)  "<PT:Motor1:Trq>"
  Bus Selector2/3 -> Subsystem1/6(MMotorRL)  "<PT:Motor2:Trq>"
  Bus Selector2/4 -> Subsystem1/7(MMotorRR)  "<PT:Motor3:Trq>"
  Bus Selector2/9 -> Subsystem1/12(PMeasured)  "<PT:PwrSupply:HV1:Pwr>"
  Constant11/1 -> Subsystem1/14(BMeasuredEnable)
  Constant12/1 -> Subsystem1/15(FF_TC)
  Constant13/1 -> Subsystem1/18(rRegenSplitF)
  Bus Selector2/5 -> Subsystem1/27(nMotorFL)  "<PT:Motor:rotv>"
  Bus Selector2/6 -> Subsystem1/28(nMotorFR)  "<PT:Motor1:rotv>"
  Bus Selector2/7 -> Subsystem1/29(nMotorRL)  "<PT:Motor2:rotv>"
  Bus Selector2/8 -> Subsystem1/30(nMotorRR)  "<PT:Motor3:rotv>"
  Constant14/1 -> Subsystem1/24(P_PC)
  Constant15/1 -> Subsystem1/25(D_PC)
  Constant16/1 -> Subsystem1/17(rLimitHigh)
  Constant17/1 -> Subsystem1/20(rLimitLow)

== system TorqueVect/CarMaker/IPG Vehicle/PowerTrain/PTControl Example/PTControl_TC_MFE ==
  VhclCtrl.PT : Inport
  SyncIn : Inport  Port=2
  Bus Selector : BusSelector  OutputSignals=VhclCtrl Gas
  Bus Selector1 : BusSelector  OutputSignals=Vel_B x
  Bus Selector2 : BusSelector  OutputSignals=PT:Motor.PT:Motor:rotv,PT:Motor.PT:Motor1:rotv,PT:Motor.PT:Motor2:rotv,PT:Motor.PT:Motor3:rotv
  Constant : Constant
  Constant1 : Constant  Value=.5
  Constant10 : Constant  Value=21
  Constant2 : Constant  Value=0.1
  Constant5 : Constant
  Constant6 : Constant  Value=100
  Constant7 : Constant  Value=10
  Constant8 : Constant  Value=-100
  Constant9 : Constant  Value=7
  Gain{,1..3} (4 alike) : Gain  Gain=1/21
  Gain4 : Gain  Gain=3.6
  Inertial Sensor : CarMaker4SL/Sensors/Inertial Sensor  xname=Param_B00  xstime=Continuous
      settings: SourceProductName=CarMaker4SL
  Mux{,1..3} (4 alike) : Mux  Inputs=3
  NOTSET1 : Constant  Value=-99999
  NOTSET3 : Constant  Value=-99999
  New TC : Subsystem  Commented=on
  PTC : Subsystem
  Scope : Scope
  TC : Subsystem
  Terminator : Terminator
  PTC MiscOut : Outport  VectorParamsAs1DForOutWhenUnconnected=off
  MotorOut0 : Outport  Port=2  VectorParamsAs1DForOutWhenUnconnected=off
  MotorOut1 : Outport  Port=3  VectorParamsAs1DForOutWhenUnconnected=off
  MotorOut2 : Outport  Port=4  VectorParamsAs1DForOutWhenUnconnected=off
  MotorOut3 : Outport  Port=5  VectorParamsAs1DForOutWhenUnconnected=off
  wires:
  VhclCtrl.PT/1 -> Bus Selector/1
  PTC/1(PTC MiscOut) -> PTC MiscOut/1
  Inertial Sensor/2 -> Bus Selector1/1
  Bus Selector1/1 -> TC/2(vLong), Gain4/1  "<Vel_B x>"
  Inertial Sensor/1 -> Terminator/1
  Mux/1 -> MotorOut0/1
  Mux3/1 -> MotorOut3/1
  Mux2/1 -> MotorOut2/1
  Mux1/1 -> MotorOut1/1
  NOTSET3/1 -> Mux3/2, Mux1/2, Mux/2, Mux2/2
  NOTSET1/1 -> Mux/3, Mux1/3, Mux2/3, Mux3/3  "rotv_trg"
  Gain/1 -> Mux/1
  Gain1/1 -> Mux1/1
  Gain2/1 -> Mux2/1
  Gain3/1 -> Mux3/1
  Gain4/1 -> Scope/1
  SyncIn/1 -> Bus Selector2/1
  TC/1(MMotorDemandFL) -> Gain/1
  TC/2(MMotorDemandFR) -> Gain1/1
  TC/3(MMotorDemandRL) -> Gain2/1
  TC/4(MMotorDemandRR) -> Gain3/1
  Bus Selector/1 -> TC/1(rThrottlePedal)  "<VhclCtrl Gas>"
  Constant1/1 -> TC/7(rSplitF)
  Constant10/1 -> TC/8(MMotorMax)
  Constant2/1 -> TC/10(rSlipTargetR), TC/9(rSlipTargetF)
  Constant/1 -> TC/11(BEnableTC)
  Constant7/1 -> TC/12(P_TC)
  Constant9/1 -> TC/13(D_TC)
  Constant5/1 -> TC/14(FF_TC)
  Constant6/1 -> TC/15(rLimitHigh)
  Constant8/1 -> TC/16(rLimitLow)
  Bus Selector2/1 -> TC/3(nMotorFL)  "<PT:Motor:rotv>"
  Bus Selector2/2 -> TC/4(nMotorFR)  "<PT:Motor1:rotv>"
  Bus Selector2/3 -> TC/5(nMotorRL)  "<PT:Motor2:rotv>"
  Bus Selector2/4 -> TC/6(nMotorRR)  "<PT:Motor3:rotv>"

== system TorqueVect/CarMaker/IPG Vehicle/PowerTrain/PTControl Example/PTControl_TV_IPG ==
  note: Minimalistic PTControl
      | example model
      | to be used with
      | FSE_TorqueVectoring
  VhclCtrl.PT : Inport
  Bus Selector : BusSelector  OutputSignals=VhclCtrl Gas
  PTC : Subsystem
  Torque Control 0 : Subsystem
  Torque Control 1 : Subsystem
  Torque Control 2 : Subsystem
  Torque Control 3 : Subsystem
  PTC MiscOut : Outport  VectorParamsAs1DForOutWhenUnconnected=off
  MotorOut0 : Outport  Port=2  VectorParamsAs1DForOutWhenUnconnected=off
  MotorOut1 : Outport  Port=3  VectorParamsAs1DForOutWhenUnconnected=off
  MotorOut2 : Outport  Port=4  VectorParamsAs1DForOutWhenUnconnected=off
  MotorOut3 : Outport  Port=5  VectorParamsAs1DForOutWhenUnconnected=off
  wires:
  Bus Selector/1 -> Torque Control 1/1(Gas), Torque Control 0/1(Gas), Torque Control 3/1(Gas), Torque Control 2/1(Gas)  "<VhclCtrl Gas>"
  Torque Control 3/1(MotorOut3) -> MotorOut3/1
  Torque Control 2/1(MotorOut2) -> MotorOut2/1
  Torque Control 1/1(MotorOut1) -> MotorOut1/1
  VhclCtrl.PT/1 -> Bus Selector/1
  Torque Control 0/1(MotorOut0) -> MotorOut0/1
  PTC/1(PTC MiscOut) -> PTC MiscOut/1

== system TorqueVect/CarMaker/IPG Vehicle/PowerTrain/PTControl Example/PTControl_TV_MFE1 ==
  VhclCtrl.PT : Inport
  SyncIn : Inport  Port=2
  Bus Selector : BusSelector  OutputSignals=VhclCtrl Brake,VhclCtrl Gas
  Bus Selector1 : BusSelector  OutputSignals=Vel_B x,Vel_B y
  Bus Selector2 : BusSelector  OutputSignals=Driver:Steer:Ang
  Constant : Constant
  Constant1 : Constant  Value=0.4
  Constant10 : Constant  Value=21
  Constant11 : Constant  Value=0.4
  Constant12 : Constant  Value=15
  Constant2 : Constant  Value=2
  Constant3 : Constant  Value=0.07
  Constant4 : Constant  Value=2
  Constant5 : Constant  Value=0.33
  Constant7 : Constant  Value=10
  Constant9 : Constant  Value=0.5
  Gain{,1..3} (4 alike) : Gain  Gain=1/21
  Gain4 : Gain  Gain=3.6
  Inertial Sensor : CarMaker4SL/Sensors/Inertial Sensor  xname=Param_B00  xstime=Continuous
      settings: SourceProductName=CarMaker4SL
  Mux{,1..3} (4 alike) : Mux  Inputs=3
  NOTSET1 : Constant  Value=-99999
  NOTSET3 : Constant  Value=-99999
  New TC : Subsystem  Commented=on
  PTC : Subsystem
  Scope : Scope
  Subsystem : Subsystem
  Terminator : Terminator
  PTC MiscOut : Outport  VectorParamsAs1DForOutWhenUnconnected=off
  MotorOut0 : Outport  Port=2  VectorParamsAs1DForOutWhenUnconnected=off
  MotorOut1 : Outport  Port=3  VectorParamsAs1DForOutWhenUnconnected=off
  MotorOut2 : Outport  Port=4  VectorParamsAs1DForOutWhenUnconnected=off
  MotorOut3 : Outport  Port=5  VectorParamsAs1DForOutWhenUnconnected=off
  wires:
  VhclCtrl.PT/1 -> Bus Selector/1
  PTC/1(PTC MiscOut) -> PTC MiscOut/1
  Inertial Sensor/2 -> Bus Selector1/1
  Bus Selector1/1 -> Subsystem/1(vLong), Gain4/1  "<Vel_B x>"
  Inertial Sensor/1 -> Terminator/1
  Mux/1 -> MotorOut0/1
  Mux3/1 -> MotorOut3/1
  Mux2/1 -> MotorOut2/1
  Mux1/1 -> MotorOut1/1
  NOTSET3/1 -> Mux3/2, Mux1/2, Mux/2, Mux2/2
  NOTSET1/1 -> Mux/3, Mux1/3, Mux2/3, Mux3/3  "rotv_trg"
  Gain/1 -> Mux/1
  Gain1/1 -> Mux1/1
  Gain2/1 -> Mux2/1
  Gain3/1 -> Mux3/1
  Gain4/1 -> Scope/1
  SyncIn/1 -> Bus Selector2/1
  Subsystem/1(NTorqueLeftOut) -> Gain/1
  Subsystem/2(NTorqueRightOut) -> Gain1/1
  Subsystem/3(NTorqueLeftOut1) -> Gain2/1
  Subsystem/4(NTorqueRightOut1) -> Gain3/1
  Bus Selector/2 -> Subsystem/12(rThrottle)  "<VhclCtrl Gas>"
  Constant1/1 -> Subsystem/7(rSplitF)
  Constant10/1 -> Subsystem/13(MMotorMax)
  Constant/1 -> Subsystem/6(BTorqueVectoringEnable)
  Constant7/1 -> Subsystem/8(P_YR)
  Constant9/1 -> Subsystem/9(D_YR)
  Constant5/1 -> Subsystem/15(rSteerWheel)
  Constant2/1 -> Subsystem/3(vLongMin)
  Constant3/1 -> Subsystem/4(aSteerWheelMin)
  Constant4/1 -> Subsystem/5(NTorqueMaxDeltaF)
  Constant11/1 -> Subsystem/10(rRegenSplitF)
  Constant12/1 -> Subsystem/16(NTorqueMaxDeltaR)
  Bus Selector/1 -> Subsystem/11(NBrake)  "<VhclCtrl Brake>"
  Bus Selector1/2 -> Subsystem/14(vLat)  "<Vel_B y>"
  Bus Selector2/1 -> Subsystem/2(aSteerWheel)  "<Driver:Steer:Ang>"

== system TorqueVect/CarMaker/IPG Vehicle/PowerTrain/PTControl Example/PTControl_TV_MFE2 ==
  VhclCtrl.PT : Inport
  SyncIn : Inport  Port=2
  Bus Selector : BusSelector  OutputSignals=VhclCtrl Brake,VhclCtrl Gas
  Bus Selector1 : BusSelector  OutputSignals=Vel_B x,Vel_B y
  Bus Selector2 : BusSelector  OutputSignals=Steer.Driver:Steer:Ang
  Constant : Constant
  Constant10 : Constant  Value=21
  Constant12 : Constant  Value=15
  Constant2 : Constant  Value=2
  Constant3 : Constant  Value=0.07
  Constant4 : Constant  Value=2
  Constant5 : Constant  Value=0.33
  Constant7 : Constant  Value=10
  Constant9 : Constant  Value=0.5
  Gain{,1..3} (4 alike) : Gain  Gain=1/21
  Gain4 : Gain  Gain=3.6
  Inertial Sensor : CarMaker4SL/Sensors/Inertial Sensor  xname=Param_B00  xstime=Continuous
      settings: SourceProductName=CarMaker4SL
  Mux{,1..4} (5 alike) : Mux  Inputs=3
  NOTSET1 : Constant  Value=-99999
  NOTSET3 : Constant  Value=-99999
  New TC : Subsystem  Commented=on
  PTC : Subsystem
  Scope : Scope
  Subsystem : Subsystem
  Terminator : Terminator
  PTC MiscOut : Outport  VectorParamsAs1DForOutWhenUnconnected=off
  MotorOut0 : Outport  Port=2  VectorParamsAs1DForOutWhenUnconnected=off
  MotorOut1 : Outport  Port=3  VectorParamsAs1DForOutWhenUnconnected=off
  MotorOut2 : Outport  Port=4  VectorParamsAs1DForOutWhenUnconnected=off
  MotorOut3 : Outport  Port=5  VectorParamsAs1DForOutWhenUnconnected=off
  a|Slip : Outport  Port=6
  wires:
  VhclCtrl.PT/1 -> Bus Selector/1
  PTC/1(PTC MiscOut) -> PTC MiscOut/1
  Inertial Sensor/2 -> Bus Selector1/1
  Bus Selector1/1 -> Subsystem/1(vLong), Gain4/1  "<Vel_B x>"
  Inertial Sensor/1 -> Terminator/1
  Mux/1 -> MotorOut0/1
  Mux3/1 -> MotorOut3/1
  Mux2/1 -> MotorOut2/1
  Mux1/1 -> MotorOut1/1
  NOTSET3/1 -> Mux3/2, Mux1/2, Mux/2, Mux2/2, Mux4/1
  NOTSET1/1 -> Mux/3, Mux1/3, Mux2/3, Mux3/3, Mux4/3  "rotv_trg"
  Gain/1 -> Mux/1
  Gain1/1 -> Mux1/1
  Gain2/1 -> Mux2/1
  Gain3/1 -> Mux3/1
  Gain4/1 -> Scope/1
  SyncIn/1 -> Bus Selector2/1
  Subsystem/1(NTorqueLeftOut) -> Gain/1
  Subsystem/2(NTorqueRightOut) -> Gain1/1
  Subsystem/3(NTorqueLeftOut1) -> Gain2/1
  Subsystem/4(NTorqueRightOut1) -> Gain3/1
  Bus Selector/2 -> Subsystem/10(rThrottle)  "<VhclCtrl Gas>"
  Constant10/1 -> Subsystem/11(MMotorMax)
  Constant/1 -> Subsystem/6(BTorqueVectoringEnable)
  Constant7/1 -> Subsystem/7(P_YR)
  Constant9/1 -> Subsystem/8(D_YR)
  Constant5/1 -> Subsystem/13(rSteerWheel)
  Constant2/1 -> Subsystem/3(vLongMin)
  Constant3/1 -> Subsystem/4(aSteerWheelMin)
  Constant4/1 -> Subsystem/5(NTorqueMaxDeltaF)
  Constant12/1 -> Subsystem/14(NTorqueMaxDeltaR)
  Bus Selector/1 -> Subsystem/9(NBrake)  "<VhclCtrl Brake>"
  Bus Selector1/2 -> Subsystem/12(vLat)  "<Vel_B y>"
  Bus Selector2/1 -> Subsystem/2(aSteerWheel)  "<Driver:Steer:Ang>"
  Mux4/1 -> a|Slip/1
  Subsystem/5(aSlip) -> Mux4/2

== system TorqueVect/CarMaker/IPG Vehicle/PowerTrain/PTControl Example/PTControl_TV_MFE25 ==
  VhclCtrl.PT : Inport
  SyncIn : Inport  Port=2
  Bus Selector : BusSelector  OutputSignals=VhclCtrl Brake,VhclCtrl Gas
  Bus Selector1 : BusSelector  OutputSignals=Vel_B x,Vel_B y
  Bus Selector2 : BusSelector  OutputSignals=Steer.Driver:Steer:Ang,PT:Motor.PT:Motor:rotv,PT:Motor.PT:Motor1:rotv,PT:Motor.PT:Motor2:rotv,PT:Motor.PT:Motor3:rotv
  Constant1 : Constant  Value=.5
  Constant10 : Constant  Value=.7
  Constant2 : Constant  Value=0
  Constant3 : Constant  Value=0
  Constant4 : Constant  Value=0.1
  Constant7 : Constant  Value=80000
  Constant9 : Constant  Value=21
  Define XcpTorqueActive : CarMaker4SL/Define CM Dict  xname=TorqueVect.XcpTorqueActive  xunit=-  xmono=off  xtype=UChar  xdvaplace=None  xnstates=2  xfirststate=0  xinitial=0
  Define XcpTorqueRequestNm : CarMaker4SL/Define CM Dict  xname=TorqueVect.XcpTorqueRequestNm  xunit=N.m  xmono=off  xtype=Double  xdvaplace=None  xnstates=0  xfirststate=0  xinitial=0
  Full Control Loop : Subsystem
  Gain{,1..3} (4 alike) : Gain  Gain=1/21
  Gain4 : Gain  Gain=3.6
  Inertial Sensor : CarMaker4SL/Sensors/Inertial Sensor  xname=Param_B00  xstime=Continuous
      settings: SourceProductName=CarMaker4SL
  Multiply : Gain  Gain=2*pi/60
  Mux{,1..4} (5 alike) : Mux  Inputs=3
  Mux5 : Mux
  Mux6 : Mux
  NOTSET1 : Constant  Value=-99999
  NOTSET3 : Constant  Value=-99999
  New TC : Subsystem  Commented=on
  PTC : Subsystem
  Read XcpTorqueActive : CarMaker4SL/Read CM Dict  xname=MFE_CAN.DriveActive  xsync=on  xstime=Continuous
  Read XcpTorqueRequestNm : CarMaker4SL/Read CM Dict  xname=MFE_CAN.TorqueRequestTotalNm  xsync=on  xstime=Continuous
  Scope : Scope
  Terminator : Terminator
  XcpTorque to u : Gain  Gain=1/(4*T_i_max)
  u Source Switch : Switch  Criteria=u2 ~= 0  SaturateOnIntegerOverflow=off  InputSameDT=off
  PTC MiscOut : Outport  VectorParamsAs1DForOutWhenUnconnected=off
  MotorOut0 : Outport  Port=2  VectorParamsAs1DForOutWhenUnconnected=off
  MotorOut1 : Outport  Port=3  VectorParamsAs1DForOutWhenUnconnected=off
  MotorOut2 : Outport  Port=4  VectorParamsAs1DForOutWhenUnconnected=off
  MotorOut3 : Outport  Port=5  VectorParamsAs1DForOutWhenUnconnected=off
  a|Slip : Outport  Port=6
  wires:
  VhclCtrl.PT/1 -> Bus Selector/1
  PTC/1(PTC MiscOut) -> PTC MiscOut/1
  Inertial Sensor/2 -> Bus Selector1/1
  Bus Selector1/1 -> Full Control Loop/5(vehicle_speed), Gain4/1  "<Vel_B x>"
  Inertial Sensor/1 -> Terminator/1
  Mux/1 -> MotorOut0/1
  Mux3/1 -> MotorOut3/1
  Mux2/1 -> MotorOut2/1
  Mux1/1 -> MotorOut1/1
  NOTSET3/1 -> Mux3/2, Mux1/2, Mux/2, Mux2/2, Mux4/1
  NOTSET1/1 -> Mux/3, Mux1/3, Mux2/3, Mux3/3, Mux4/3  "rotv_trg"
  Gain/1 -> Mux/1
  Gain1/1 -> Mux1/1
  Gain2/1 -> Mux2/1
  Gain3/1 -> Mux3/1
  Gain4/1 -> Scope/1
  SyncIn/1 -> Bus Selector2/1
  Full Control Loop/1(\tau_1) -> Gain/1
  Full Control Loop/2(\tau_2) -> Gain1/1
  Full Control Loop/3(\tau_3) -> Gain2/1
  Full Control Loop/4(\tau_4) -> Gain3/1
  Constant10/1 -> Full Control Loop/11(efficiency)
  Constant7/1 -> Full Control Loop/7(P_max)
  Constant9/1 -> Full Control Loop/8(T_i_max)
  Constant2/1 -> Full Control Loop/1(l_lim)
  Constant3/1 -> Full Control Loop/2(ResetSignal)
  Constant4/1 -> Full Control Loop/6(min_speed)
  Mux4/1 -> a|Slip/1
  [TireFL] -> Mux5/1
  [TireFR] -> Mux5/2
  [TireRL] -> Mux5/3
  [TireRR] -> Mux5/4
  Mux5/1 -> Full Control Loop/4(Fz_per_wheel)
  Constant1/1 -> Full Control Loop/9(lamda)
  Bus Selector2/2 -> Mux6/1  "<PT:Motor:rotv>"
  Bus Selector2/3 -> Mux6/2  "<PT:Motor1:rotv>"
  Bus Selector2/4 -> Mux6/3  "<PT:Motor2:rotv>"
  Bus Selector2/5 -> Mux6/4  "<PT:Motor3:rotv>"
  Mux6/1 -> Multiply/1
  Multiply/1 -> Full Control Loop/10(omega)
  Read XcpTorqueRequestNm/1 -> XcpTorque to u/1
  XcpTorque to u/1 -> u Source Switch/1
  Read XcpTorqueActive/1 -> u Source Switch/2
  Bus Selector/2 -> u Source Switch/3  "<VhclCtrl Gas>"
  u Source Switch/1 -> Full Control Loop/3(u)
